simulink model "PlanarRobot5link"  (R2022b)
settings: Solver=VariableStepAuto  StartTime=0.0  StopTime=30  RelTol=1e-3
values from neighbouring files (symbols this model uses):
  I = [1; 1; 1; 0.5; 0.5]*0.2    [RobDyn4link.m]
  l = [1; 1; 1; 1; 2]*0.2    [RobDyn4link.m]
  lc = l./2    [RobDyn4link.m]
  m = [1; 1; 1; 0.3; 0.3]*1    [RobDyn4link.m]
  q0 = [pi/2; -pi/4; -1*pi/6;-pi/12;0;]    [RobDyn4link.m]
  theta_max = [0.915*pi; 0.915*pi; 0.915*pi; 0.915*pi; 0.915*pi;]    [RobDyn4link.m]
  theta_min = [-0.915*pi; -0.915*pi; -0.915*pi; -0.915*pi; -0.915*pi;]    [RobDyn4link.m]
libraries: slpidlib x1
(part 1 of 3)
settings Model: Creator=yu  LastModifiedBy=yu

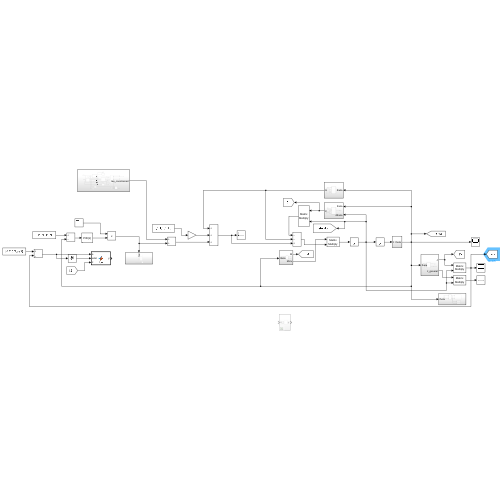
[thumbnail: Simulink's stored preview of the top-level diagram]
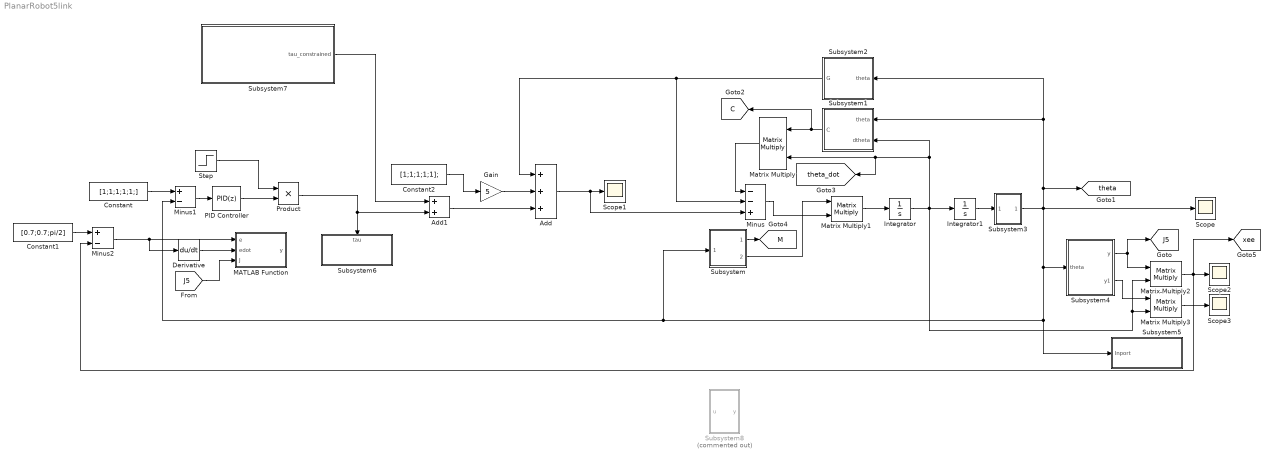
== system PlanarRobot5link ==
  Add : Sum  Inputs=+++
  Add1 : Sum
  Constant : Constant  Value=[1;1;1;1;1;]
  Constant1 : Constant  Value=[0.7;0.7;pi/2]
  Constant2 : Constant  Value=[1;1;1;1;1];
  Derivative : Derivative
  Gain : Gain  Gain=5
  Integrator : Integrator
  Integrator1 : Integrator  InitialCondition=q0
  MATLAB Function : MATLAB Function  TreatAsAtomicUnit=on
  Matrix Multiply{,1..3} (4 alike) : Product  Multiplication=Matrix(*)
  Minus : Sum  Inputs=--+
  Minus1 : Sum  Inputs=+-
  Minus2 : Sum  Inputs=+-
  PID Controller : slpidlib/PID Controller  Controller=PID  Form=Parallel  TimeDomain=Discrete-time  UseExternalTs=off  SampleTime=1e-3  IntegratorMethod=Forward Euler  FilterMethod=Forward Euler  ControllerParametersSource=internal  P=5  I=0  UseKiTs=off  D=1  N=100  UseFilter=on  TunerSelectOption=Transfer Function Based (PID Tuner App)  InitialConditionSource=internal  InitialConditionForIntegrator=0  InitialConditionForFilter=0  DifferentiatorICPrevScaledInput=0  ExternalReset=none  TrackingMode=off  Kt=1  LimitOutput=off  SatLimitsSource=internal  UpperSaturationLimit=inf  LowerSaturationLimit=-inf  LinearizeAsGain=on  AntiWindupMode=none  Kb=1  LimitIntegrator=off  UpperIntegratorSaturationLimit=inf  LowerIntegratorSaturationLimit=-inf  POutMin=[]  POutMax=[]  IOutMin=[]  IOutMax=[]  DOutMin=[]  DOutMax=[]  NOutMin=[]  NOutMax=[]  SumOutMin=[]  SumOutMax=[]  SaturationOutMin=[]  SaturationOutMax=[]  PParamMin=[]  PParamMax=[]  IParamMin=[]  IParamMax=[]  DParamMin=[]  DParamMax=[]  NParamMin=[]  NParamMax=[]  KbParamMin=[]  KbParamMax=[]  KtParamMin=[]  KtParamMax=[]  KbOutMin=[]  KbOutMax=[]  KtOutMin=[]  KtOutMax=[]  IntegratorOutMin=[]  IntegratorOutMax=[]  FilterOutMin=[]  FilterOutMax=[]  SumI1OutMin=[]  SumI1OutMax=[]  SumI2OutMin=[]  SumI2OutMax=[]  SumI3OutMin=[]  SumI3OutMax=[]  SumI4OutMin=[]  SumI4OutMax=[]  SumDOutMin=[]  SumDOutMax=[]  DifferentiatorOutMin=[]  DifferentiatorOutMax=[]  FilterDiffOutCoefMin=[]  FilterDiffOutCoefMax=[]  ReciprocalOutMin=[]  ReciprocalOutMax=[]  SumDenOutMin=[]  SumDenOutMax=[]  SumNumOutMin=[]  SumNumOutMax=[]  DivideOutMin=[]  DivideOutMax=[]  UdiffTsProdOutMin=[]  UdiffTsProdOutMax=[]  NTsProdOutMin=[]  NTsProdOutMax=[]  UintegralTsProdOutMin=[]  UintegralTsProdOutMax=[]  UngainTsProdOutMin=[]  UngainTsProdOutMax=[]  ClampingZeroOutDataTypeStr=Inherit: Inherit via back propagation  ClampingZeroOutMin=[]  ClampingZeroOutMax=[]  FilterDenConstantOutDataTypeStr=Inherit: Inherit via back propagation  FilterDenConstantOutMin=[]  FilterDenConstantOutMax=[]  PCopyOutDataTypeStr=Inherit: Inherit via back propagation  PCopyOutMin=[]  PCopyOutMax=[]  NCopyOutDataTypeStr=Inherit: Inherit via back propagation  NCopyOutMin=[]  NCopyOutMax=[]  IntegratorContinuousStateAttributes=''  IntegratorStateMustResolveToSignalObject=off  IntegratorRTWStateStorageClass=Auto  FilterContinuousStateAttributes=''  FilterStateMustResolveToSignalObject=off  FilterRTWStateStorageClass=Auto  ParallelPVariant=InternalParameters  IdealPVariant=Disabled  IVariant=InternalParameters  DVariant=InternalParameters  IntegratorVariant=Discrete  SatVariant=Disabled  AWVariant=Passthrough  PCopyVariant=Disabled  TRVariant=Disabled  FdbkBlocksVariant=Forward  IdealPFdbkVariant=Disabled  SatFdbkVariant=Disabled  DerivativeFilterVariant=ForwardEulerFilter  NVariant=InternalParameters  NCopyVariant=Disabled  FilterICVariant=InternalICsFilter  IntegratorICVariant=InternalICs  ExternalResetVariant=Disabled  TRSumVariant=Passthrough  SumFdbkVariant=Disabled  SumVariant=Sum_PID  TsampFilterVariant=InternalTs  TsampNgainVariant=Passthrough  TsampIntegralVariant=Passthrough  ExternalSaturationOutDataTypeStr=Inherit: Same as second input
  Product : Product
  Scope{,1..3} (4 alike) : Scope
  Step : Step  Time=15  Before=1  After=0.1  SampleTime=0
  Subsystem : Subsystem
  Subsystem1 : Subsystem
  Subsystem2 : Subsystem
  Subsystem3 : Subsystem
  Subsystem4 : Subsystem
  Subsystem5 : Subsystem
  Subsystem6 : Subsystem
      settings: PortSchema="{\"entries\":[{\"content\":{\"sides\":[{\"content\":{\"connectorIds\":[]},\"type\":\"ConnectorPlacement.EquallySpacedRectSide\",\"uuid\":\"f7fb76f5-7827-4aaa-b7a2-74cca6779f28\"},{\"content\":{\"connectorIds\":[],\"side\":\"RIGHT\"},\"type\":\"ConnectorPlacement.EquallySpacedRectSide\",\"uuid\":\"f7fd9930-b971-4267-b147-daf226bd5956\"},{\"content\":{\"connectorIds\":[],\"side\":\"TOP\"},\"type\":\"ConnectorPlacement.EquallySpacedRectSide\",\"uuid\":\"712bf0c7-edba-496e-8848-dfa7514e65ee\"},{\"content\":{\"connectorIds\":[\"In1\"],\"side\":\"BOTTOM\"},\"type\":\"ConnectorPlacement.EquallySpacedRectSide\",\"uuid\":\"1940cde7-8882-437d-977e-a5c0cec78ee9\"}]},\"type\":\"ConnectorPlacement.EquallySpacedConnector\",\"uuid\":\"5c054d3d-b8b3-446f-b900-5a57edebfb92\"}],\"packageUris\":[\"http://schema.mathworks.com/mf0/Connector/R2020b\"],\"version\":\"1.0\"}"
  Subsystem7 : Subsystem
  Subsystem8 : Subsystem  Commented=on
  tag scope: C=global, J5=global, M=global, theta=global, theta_dot=global, xee=global
  wires:
  Subsystem/2(Outport1) -> Matrix Multiply1/1
  Matrix Multiply1/1 -> Integrator/1
  Minus/1 -> Matrix Multiply1/2
  Subsystem3/1(theta) -> Subsystem4/1(theta), Subsystem5/1(Inport), Minus1/2, Subsystem/1(Inport), Subsystem1/1(theta), Subsystem2/1(theta), [theta], Scope/1
  Subsystem1/1(C) -> [C], Matrix Multiply/1
  Integrator1/1 -> Subsystem3/1(In1)
  Constant/1 -> Minus1/1
  Add/1 -> Minus/3, Scope1/1
  Subsystem2/1(G) -> Add/1, Minus/2
  Matrix Multiply/1 -> Minus/1
  Minus1/1 -> PID Controller/1
  Matrix Multiply2/1 -> Minus2/2, [xee], Scope2/1
  Subsystem4/1(y) -> Matrix Multiply2/1, [J5]
  Constant1/1 -> Minus2/1
  [J5] -> MATLAB Function/3(J)
  Derivative/1 -> MATLAB Function/2(edot)
  Minus2/1 -> MATLAB Function/1(e), Derivative/1
  Add1/1 -> Add/3
  Subsystem4/2(y1) -> Matrix Multiply3/1
  Integrator/1 -> Matrix Multiply3/2, Matrix Multiply2/2, Integrator1/1, Subsystem1/2(dtheta), Matrix Multiply/2, [theta_dot]
  Matrix Multiply3/1 -> Scope3/1
  Subsystem7/1(tau_constrained) -> Add1/1
  Product/1 -> Add1/2, Subsystem6/1(tau)
  Subsystem/1(Outport) -> [M]
  PID Controller/1 -> Product/2
  Gain/1 -> Add/2
  Constant2/1 -> Gain/1
  Step/1 -> Product/1

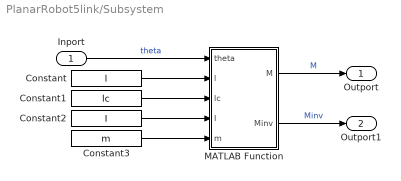
== system PlanarRobot5link/Subsystem ==
  Inport : Inport  PortDimensions=[5,1]
  Constant : Constant  Value=l
  Constant1 : Constant  Value=lc
  Constant2 : Constant  Value=I
  Constant3 : Constant  Value=m
  MATLAB Function : MATLAB Function  TreatAsAtomicUnit=on
  Outport : Outport  PortDimensions=[5,5]
  Outport1 : Outport  Port=2  PortDimensions=[5,5]
  wires:
  Constant3/1 -> MATLAB Function/5(m)
  MATLAB Function/1(M) -> Outport/1  "M"
  Inport/1 -> MATLAB Function/1(theta)  "theta"
  Constant2/1 -> MATLAB Function/4(I)
  Constant/1 -> MATLAB Function/2(l)
  Constant1/1 -> MATLAB Function/3(lc)
  MATLAB Function/2(Minv) -> Outport1/1  "Minv"

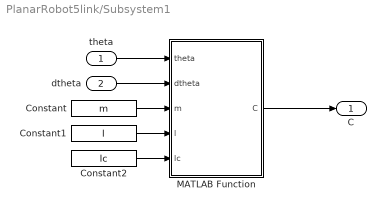
== system PlanarRobot5link/Subsystem1 ==
  theta : Inport  PortDimensions=[5,1]
  dtheta : Inport  Port=2  PortDimensions=[5,1]
  Constant : Constant  Value=m
  Constant1 : Constant  Value=l
  Constant2 : Constant  Value=lc
  MATLAB Function : MATLAB Function  TreatAsAtomicUnit=on
  C : Outport  PortDimensions=[5,5]
  wires:
  theta/1 -> MATLAB Function/1(theta)
  MATLAB Function/1(C) -> C/1
  dtheta/1 -> MATLAB Function/2(dtheta)
  Constant/1 -> MATLAB Function/3(m)
  Constant2/1 -> MATLAB Function/5(lc)
  Constant1/1 -> MATLAB Function/4(l)

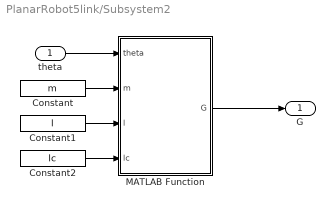
== system PlanarRobot5link/Subsystem2 ==
  theta : Inport  PortDimensions=[5,1]
  Constant : Constant  Value=m
  Constant1 : Constant  Value=l
  Constant2 : Constant  Value=lc
  MATLAB Function : MATLAB Function  TreatAsAtomicUnit=on
  G : Outport  PortDimensions=[5,1]
  wires:
  Constant1/1 -> MATLAB Function/3(l)
  Constant2/1 -> MATLAB Function/4(lc)
  Constant/1 -> MATLAB Function/2(m)
  MATLAB Function/1(G) -> G/1
  theta/1 -> MATLAB Function/1(theta)

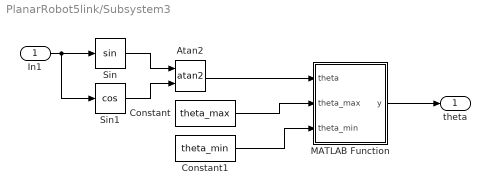
== system PlanarRobot5link/Subsystem3 ==
  In1 : Inport
  Atan2 : Trigonometry  Operator=atan2
  Constant : Constant  Value=theta_max
  Constant1 : Constant  Value=theta_min
  MATLAB Function : MATLAB Function  TreatAsAtomicUnit=on
  Sin : Trigonometry
  Sin1 : Trigonometry  Operator=cos
  theta : Outport  PortDimensions=[5,1]
  wires:
  Atan2/1 -> MATLAB Function/1(theta)
  In1/1 -> Sin1/1, Sin/1
  Sin/1 -> Atan2/1
  Sin1/1 -> Atan2/2
  MATLAB Function/1(y) -> theta/1
  Constant/1 -> MATLAB Function/2(theta_max)
  Constant1/1 -> MATLAB Function/3(theta_min)

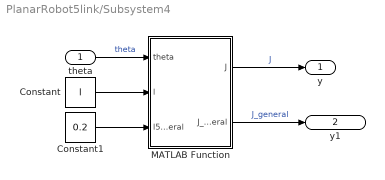
== system PlanarRobot5link/Subsystem4 ==
  theta : Inport
  Constant : Constant  Value=l
  Constant1 : Constant  Value=0.2
  MATLAB Function : MATLAB Function  TreatAsAtomicUnit=on
  y : Outport
  y1 : Outport  Port=2
  wires:
  theta/1 -> MATLAB Function/1(theta)  "theta"
  MATLAB Function/1(J) -> y/1  "J"
  Constant/1 -> MATLAB Function/2(l)
  Constant1/1 -> MATLAB Function/3(l5_general)
  MATLAB Function/2(J_general) -> y1/1  "J_general"

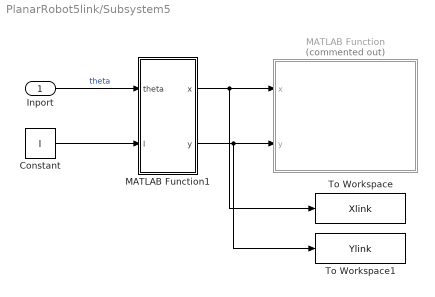
== system PlanarRobot5link/Subsystem5 ==
  Inport : Inport
  Constant : Constant  Value=l
  MATLAB Function : MATLAB Function  Commented=on  TreatAsAtomicUnit=on
  MATLAB Function1 : MATLAB Function  TreatAsAtomicUnit=on
  To Workspace : ToWorkspace  VariableName=Xlink  SaveFormat=Timeseries  SampleTime=-1
  To Workspace1 : ToWorkspace  VariableName=Ylink  SaveFormat=Timeseries  SampleTime=-1
  wires:
  MATLAB Function1/1(x) -> To Workspace/1, MATLAB Function/1(x)
  MATLAB Function1/2(y) -> To Workspace1/1, MATLAB Function/2(y)
  Inport/1 -> MATLAB Function1/1(theta)  "theta"
  Constant/1 -> MATLAB Function1/2(l)

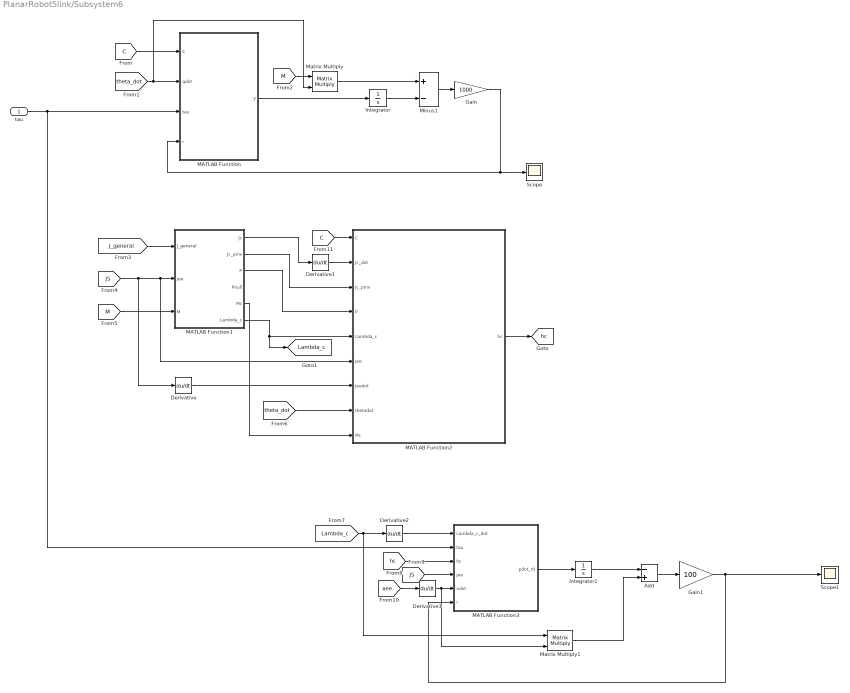
== system PlanarRobot5link/Subsystem6 ==
  tau : Inport
  Add : Sum  Inputs=-+
  Derivative{,1..3} (4 alike) : Derivative
  Gain : Gain  Gain=1000
  Gain1 : Gain  Gain=100
  Integrator : Integrator
  Integrator1 : Integrator
  MATLAB Function : MATLAB Function  TreatAsAtomicUnit=on
  MATLAB Function1 : MATLAB Function  TreatAsAtomicUnit=on
  MATLAB Function2 : MATLAB Function  TreatAsAtomicUnit=on
  MATLAB Function3 : MATLAB Function  TreatAsAtomicUnit=on
  Matrix Multiply : Product  Multiplication=Matrix(*)
  Matrix Multiply1 : Product  Multiplication=Matrix(*)
  Minus1 : Sum  Inputs=+-
  Scope : Scope
  Scope1 : Scope
  tag scope: Lambda_c=global, hc=global
  wires:
  [C] -> MATLAB Function/1(C)
  Integrator/1 -> Minus1/2
  tau/1 -> MATLAB Function3/2(tau), MATLAB Function/3(tau)
  MATLAB Function/1(y) -> Integrator/1
  [M] -> Matrix Multiply/1
  [theta_dot] -> Matrix Multiply/2, MATLAB Function/2(qdot)
  Matrix Multiply/1 -> Minus1/1
  Gain/1 -> Scope/1, MATLAB Function/4(r)
  Minus1/1 -> Gain/1
  [J_general] -> MATLAB Function1/1(J_general)
  [J5] -> MATLAB Function1/2(Jee), MATLAB Function2/6(Jee), Derivative/1
  Derivative/1 -> MATLAB Function2/7(Jeedot)
  [M] -> MATLAB Function1/3(M)
  [theta_dot] -> MATLAB Function2/8(thetadot)
  MATLAB Function1/3(P) -> MATLAB Function2/4(P)
  MATLAB Function1/2(Jc_pinv) -> MATLAB Function2/3(Jc_pinv)
  MATLAB Function1/1(Jc) -> Derivative1/1
  Derivative1/1 -> MATLAB Function2/2(Jc_dot)
  MATLAB Function1/5(Mc) -> MATLAB Function2/9(Mc)
  MATLAB Function1/6(Lambda_c) -> MATLAB Function2/5(Lambda_c), [Lambda_c]
  MATLAB Function2/1(hc) -> [hc]
  Derivative2/1 -> MATLAB Function3/1(Lambda_c_dot)
  [Lambda_c] -> Matrix Multiply1/1, Derivative2/1
  [hc] -> MATLAB Function3/3(hc)
  [J5] -> MATLAB Function3/4(Jee)
  [xee] -> Derivative3/1
  Derivative3/1 -> Matrix Multiply1/2, MATLAB Function3/5(xdot)
  MATLAB Function3/1(pdot_r0) -> Integrator1/1
  Integrator1/1 -> Add/1
  Matrix Multiply1/1 -> Add/2
  Add/1 -> Gain1/1
  Gain1/1 -> MATLAB Function3/6(r), Scope1/1
  [C] -> MATLAB Function2/1(C)

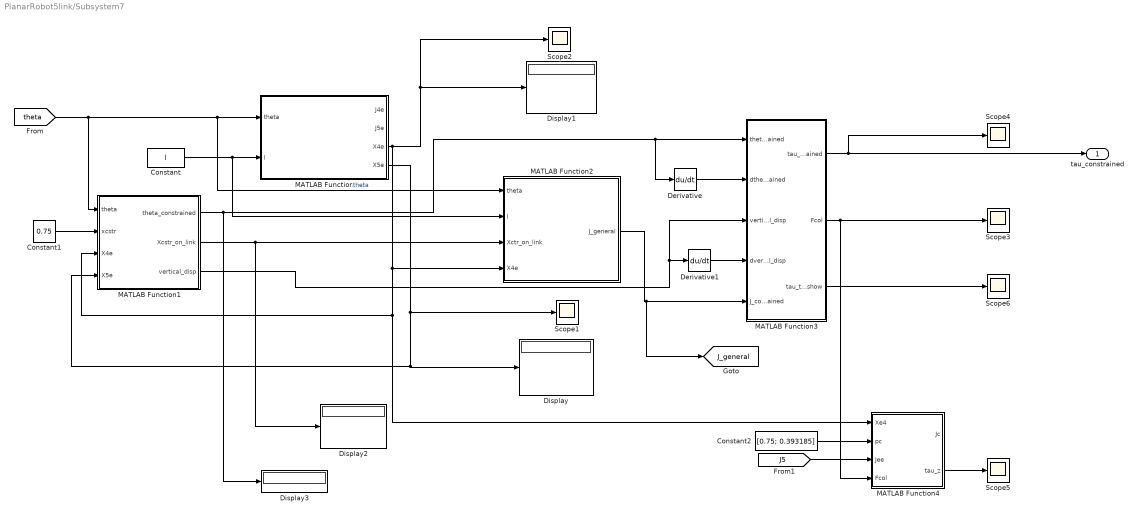
== system PlanarRobot5link/Subsystem7 ==
  Constant : Constant  Value=l
  Constant1 : Constant  Value=0.75
  Constant2 : Constant  Value=[0.75; 0.393185]
  Derivative : Derivative
  Derivative1 : Derivative
  Display{,1..3} (4 alike) : Display
  MATLAB Function : MATLAB Function  TreatAsAtomicUnit=on
  MATLAB Function1 : MATLAB Function  TreatAsAtomicUnit=on
  MATLAB Function2 : MATLAB Function  TreatAsAtomicUnit=on
  MATLAB Function3 : MATLAB Function  TreatAsAtomicUnit=on
  MATLAB Function4 : MATLAB Function  TreatAsAtomicUnit=on
  Scope{1..6} (6 alike) : Scope
  tau_constrained : Outport
  tag scope: J_general=global
  wires:
  [theta] -> MATLAB Function/1(theta), MATLAB Function2/1(theta), MATLAB Function1/1(theta)  "theta"
  Constant/1 -> MATLAB Function2/2(l), MATLAB Function/2(l)
  Constant1/1 -> MATLAB Function1/2(xcstr)
  MATLAB Function/3(X4e) -> MATLAB Function4/1(Xe4), MATLAB Function1/3(X4e), MATLAB Function2/4(X4e), Display1/1, Scope2/1
  MATLAB Function/4(X5e) -> Display/1, MATLAB Function1/4(X5e), Scope1/1
  MATLAB Function1/2(Xcstr_on_link) -> Display2/1, MATLAB Function2/3(Xctr_on_link)
  MATLAB Function2/1(J_general) -> [J_general], MATLAB Function3/5(J_constrained)
  MATLAB Function1/3(vertical_disp) -> MATLAB Function3/3(vertial_disp), Derivative1/1
  MATLAB Function1/1(theta_constrained) -> Display3/1, Derivative/1, MATLAB Function3/1(theta_constrained)
  Derivative/1 -> MATLAB Function3/2(dtheta_constrained)
  Derivative1/1 -> MATLAB Function3/4(dvertial_disp)
  MATLAB Function3/1(tau_constrained) -> Scope4/1, tau_constrained/1
  MATLAB Function3/2(Fcol) -> MATLAB Function4/4(Fcol), Scope3/1
  Constant2/1 -> MATLAB Function4/2(pc)
  [J5] -> MATLAB Function4/3(Jee)
  MATLAB Function4/2(tau_z) -> Scope5/1
  MATLAB Function3/3(tau_toshow) -> Scope6/1

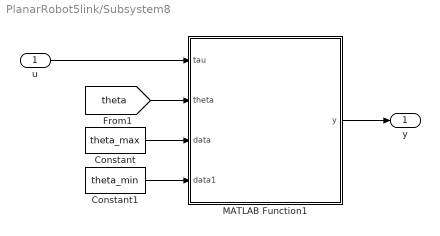
== system PlanarRobot5link/Subsystem8 ==
  u : Inport
  Constant : Constant  Value=theta_max
  Constant1 : Constant  Value=theta_min
  MATLAB Function1 : MATLAB Function  TreatAsAtomicUnit=on
  y : Outport
  wires:
  Constant1/1 -> MATLAB Function1/4(data1)
  Constant/1 -> MATLAB Function1/3(data)
  MATLAB Function1/1(y) -> y/1
  u/1 -> MATLAB Function1/1(tau)
  [theta] -> MATLAB Function1/2(theta)

== matlab function PlanarRobot5link/Subsystem7/MATLAB Function ==
  data: J4e output; J5e output; theta input; X4e output size=[3,1]; l input; X5e output size=[3,1]
function [J4e, J5e,X4e,X5e] = fcn(theta,l)

l1 = l(1); l2 = l(2); l3 = l(3); l4 = l(4); l5 = l(5);
theta1 = theta(1); theta2 = theta(2); theta3 = theta(3); theta4 = theta(4); theta5 = theta(5);

x4e = l1 * cos(theta1) + l2 * cos(theta1 + theta2) + l3 * cos(theta1 + theta2 + theta3) + l4 * cos(theta1 + theta2 + theta3 + theta4);
y4e = l1 * sin(theta1) + l2 * sin(theta1 + theta2) + l3 * sin(theta1 + theta2 + theta3) + l4 * sin(theta1 + theta2 + theta3 + theta4);
X4e = [x4e;y4e;theta1 + theta2 + theta3 + theta4];

x5e = l4*cos(theta1 + theta2 + theta3 + theta4) + l2*cos(theta1 + theta2) + l1*cos(theta1) + l5*cos(theta1 + theta2 + theta3 + theta4 + theta5) + l3*cos(theta1 + theta2 + theta3);
y5e = l4*sin(theta1 + theta2 + theta3 + theta4) + l2*sin(theta1 + theta2) + l1*sin(theta1) + l5*sin(theta1 + theta2 + theta3 + theta4 + theta5) + l3*sin(theta1 + theta2 + theta3);
X5e = [x5e;y5e;theta1 + theta2 + theta3 + theta4 + theta5];


J5e =[- l4*sin(theta1 + theta2 + theta3 + theta4) - l2*sin(theta1 + theta2) - l1*sin(theta1) - l5*sin(theta1 + theta2 + theta3 + theta4 + theta5) - l3*sin(theta1 + theta2 + theta3), - l4*sin(theta1 + theta2 + theta3 + theta4) - l2*sin(theta1 + theta2) - l5*sin(theta1 + theta2 + theta3 + theta4 + theta5) - l3*sin(theta1 + theta2 + theta3), - l4*sin(theta1 + theta2 + theta3 + theta4) - l5*sin(theta1 + theta2 + theta3 + theta4 + theta5) - l3*sin(theta1 + theta2 + theta3), - l4*sin(theta1 + theta2 + theta3 + theta4) - l5*sin(theta1 + theta2 + theta3 + theta4 + theta5), -l5*sin(theta1 + theta2 + theta3 + theta4 + theta5);
  l4*cos(theta1 + theta2 + theta3 + theta4) + l2*cos(theta1 + theta2) + l1*cos(theta1) + l5*cos(theta1 + theta2 + theta3 + theta4 + theta5) + l3*cos(theta1 + theta2 + theta3),   l4*cos(theta1 + theta2 + theta3 + theta4) + l2*cos(theta1 + theta2) + l5*cos(theta1 + theta2 + theta3 + theta4 + theta5) + l3*cos(theta1 + theta2 + theta3),   l4*cos(theta1 + theta2 + theta3 + theta4) + l5*cos(theta1 + theta2 + theta3 + theta4 + theta5) + l3*cos(theta1 + theta2 + theta3),   l4*cos(theta1 + theta2 + theta3 + theta4) + l5*cos(theta1 + theta2 + theta3 + theta4 + theta5),  l5*cos(theta1 + theta2 + theta3 + theta4 + theta5);
                                                                                                                                                                             1,                                                                                                                                                             1,                                                                                                                                   1,                                                                                                1,                                                   1;];

J4e = [- l4*sin(theta1 + theta2 + theta3 + theta4) - l2*sin(theta1 + theta2) - l1*sin(theta1) - l3*sin(theta1 + theta2 + theta3), - l4*sin(theta1 + theta2 + theta3 + theta4) - l2*sin(theta1 + theta2) - l3*sin(theta1 + theta2 + theta3), - l4*sin(theta1 + theta2 + theta3 + theta4) - l3*sin(theta1 + theta2 + theta3), -l4*sin(theta1 + theta2 + theta3 + theta4), 0;
  l4*cos(theta1 + theta2 + theta3 + theta4) + l2*cos(theta1 + theta2) + l1*cos(theta1) + l3*cos(theta1 + theta2 + theta3),   l4*cos(theta1 + theta2 + theta3 + theta4) + l2*cos(theta1 + theta2) + l3*cos(theta1 + theta2 + theta3),   l4*cos(theta1 + theta2 + theta3 + theta4) + l3*cos(theta1 + theta2 + theta3),  l4*cos(theta1 + theta2 + theta3 + theta4), 0;
                                                                                                                        1,                                                                                                        1,                                                                              1,                                          1, 0];

== matlab function PlanarRobot5link/Subsystem7/MATLAB Function1 ==
  data: theta input; theta_constrained output; xcstr input; Xcstr_on_link output; X4e input; X5e input; vertical_disp output
function [theta_constrained,Xcstr_on_link,vertical_disp] = fcn(theta,xcstr,X4e,X5e)
% theta5 = theta(5);
% % theta_constrained = atan2(X4e(2),X4e(1)) - atan2(X5e(2),X5e(1));
theta_constrained = - X5e(3);
vertical_disp = (xcstr(1)-X4e(1))/(X5e(1)-X4e(1))*(X5e(2) - X4e(2)) + X4e(2);
Xcstr_on_link = [xcstr;vertical_disp];

== matlab function PlanarRobot5link/Subsystem7/MATLAB Function2 ==
  data: theta input; J_general output; l input; Xctr_on_link input; X4e input
function J_general = fcn(theta,l,Xctr_on_link, X4e)
l5_general = sqrt((Xctr_on_link(1) - X4e(1))*(Xctr_on_link(1) - X4e(1)) + (Xctr_on_link(2) - X4e(2))*(Xctr_on_link(2) - X4e(2)));

l1 = l(1); l2 = l(2); l3 = l(3); l4 = l(4); l5 = l(5);
theta1 = theta(1); theta2 = theta(2); theta3 = theta(3); theta4 = theta(4); theta5 = theta(5);

 
J_general = [- l4*sin(theta1 + theta2 + theta3 + theta4) - l2*sin(theta1 + theta2) - l1*sin(theta1) - l5_general*sin(theta1 + theta2 + theta3 + theta4 + theta5) - l3*sin(theta1 + theta2 + theta3), - l4*sin(theta1 + theta2 + theta3 + theta4) - l2*sin(theta1 + theta2) - l5_general*sin(theta1 + theta2 + theta3 + theta4 + theta5) - l3*sin(theta1 + theta2 + theta3), - l4*sin(theta1 + theta2 + theta3 + theta4) - l5_general*sin(theta1 + theta2 + theta3 + theta4 + theta5) - l3*sin(theta1 + theta2 + theta3), - l4*sin(theta1 + theta2 + theta3 + theta4) - l5_general*sin(theta1 + theta2 + theta3 + theta4 + theta5), -l5_general*sin(theta1 + theta2 + theta3 + theta4 + theta5);
  l4*cos(theta1 + theta2 + theta3 + theta4) + l2*cos(theta1 + theta2) + l1*cos(theta1) + l5_general*cos(theta1 + theta2 + theta3 + theta4 + theta5) + l3*cos(theta1 + theta2 + theta3),   l4*cos(theta1 + theta2 + theta3 + theta4) + l2*cos(theta1 + theta2) + l5_general*cos(theta1 + theta2 + theta3 + theta4 + theta5) + l3*cos(theta1 + theta2 + theta3),   l4*cos(theta1 + theta2 + theta3 + theta4) + l5_general*cos(theta1 + theta2 + theta3 + theta4 + theta5) + l3*cos(theta1 + theta2 + theta3),   l4*cos(theta1 + theta2 + theta3 + theta4) + l5_general*cos(theta1 + theta2 + theta3 + theta4 + theta5),  l5_general*cos(theta1 + theta2 + theta3 + theta4 + theta5);
                                                                                                                                                                                     1,                                                                                                                                                                     1,                                                                                                                                           1,                                                                                                        1,                                                           1];

== matlab function PlanarRobot5link/Subsystem8/MATLAB Function1 ==
  data: tau input; y output; theta input; data input; data1 input
function y = fcn(tau, theta, data, data1)
% tau = zeros(5,1);

y = tau;

== matlab function PlanarRobot5link/Subsystem6/MATLAB Function ==
  data: C input; qdot input; y output; tau input; r input
function y = fcn(C, qdot, tau,r)

y = tau - C'*qdot + r;

== matlab function PlanarRobot5link/Subsystem7/MATLAB Function4 ==
  data: Xe4 input; Jc output; pc input; Jee input; Fcol input; tau_z output
function [Jc,tau_z] = fcn(Xe4, pc, Jee, Fcol)
pr = Xe4(1:2);
theta4 = Xe4(3);

R = [cos(theta4), -sin(theta4); sin(theta4), cos(theta4)];
y = R(:,2);
dir = pr - pc;
A = [-y(1), y(2), dir(2)*y(2) - dir(1)*y(1)];
Jc = A*Jee;

tau_z = Jc'*Fcol(2);
